simulink model "analog_filter"  (R2017b)
settings: Solver=VariableStepAuto  StartTime=0.0  StopTime=10.0  RelTol=1e-3
settings Model: Creator=Heisenberg  LastModifiedBy=Heisenberg

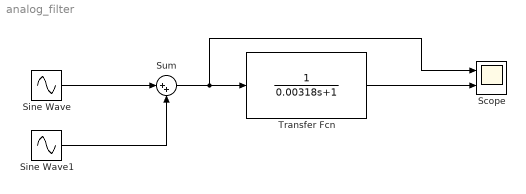
== system analog_filter ==
  Scope : Scope  NumInputPorts=2
  Sine Wave : Sin  Frequency=2*pi*50  SampleTime=0
  Sine Wave1 : Sin  Frequency=2*pi*2000  SampleTime=0
  Sum : Sum  Inputs=|++
  Transfer Fcn : TransferFcn  Denominator=[0.00318 1]
  wires:
  Sum/1 -> Scope/1, Transfer Fcn/1
  Sine Wave1/1 -> Sum/2
  Sine Wave/1 -> Sum/1
  Transfer Fcn/1 -> Scope/2
